simulink model "RETRO_IFF_NON_LIN"  (R2021a)
settings: Solver=VariableStepAuto  StartTime=0.0  StopTime=300  RelTol=1e-3
model workspace (MATLAB code in the model file):
  | Kab=14;
  | Fa=4;
  | Kba=10;
  | Fb=4;
  | Kca=8;
  | Kcb=3.2;
  | Kcd=6;
  | Fc=2;
  | Kdc=6;
  | Fd=0.5;
  | Kia=5;
  | Fa=6;
  | In=0.3;
  | x_star=[0.25;0.625;0.0833;0];
settings Model: Creator=priya  LastModifiedBy=Priyan_PC
settings SolverCC: AlgebraicLoopSolver=TrustRegion
settings DebuggingCC: SFMachineParentedDataDiag=warning

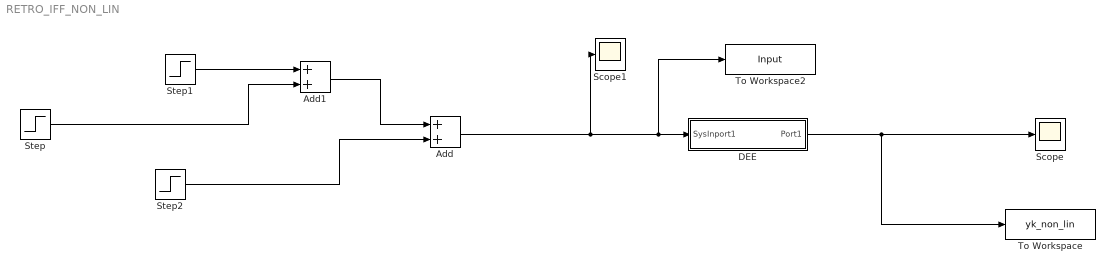
== system RETRO_IFF_NON_LIN ==
  Add : Sum
  Add1 : Sum
  DEE : Subsystem  mask(Differential Equation Editor (DEE)){}
      settings: OpenFcn=diffeqed
      mask Display: disp('Differential Equation\n Editor')
  Scope : Scope
  Scope1 : Scope
  Step : Step  Time=75  After=0.15  SampleTime=0
  Step1 : Step  Time=0  Before=0.3  After=0.5  SampleTime=0
  Step2 : Step  Time=150  After=0.15  SampleTime=0
  To Workspace : ToWorkspace  VariableName=yk_non_lin  SampleTime=-1
  To Workspace2 : ToWorkspace  VariableName=Input  SampleTime=-1
  wires:
  Step1/1 -> Add1/1
  Step/1 -> Add1/2
  Step2/1 -> Add/2
  Add1/1 -> Add/1
  Add/1 -> To Workspace2/1, DEE/1(SysInport1), Scope1/1
  DEE/1(Port1) -> To Workspace/1, Scope/1

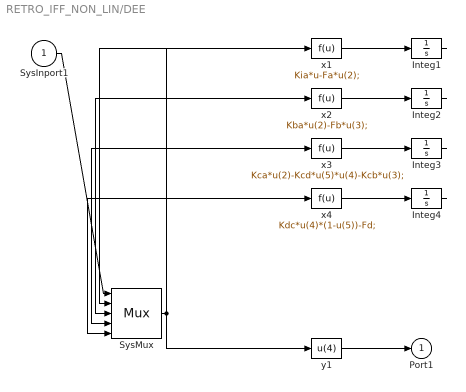
== system RETRO_IFF_NON_LIN/DEE ==
  SysInport1 : Inport
  Integ1 : Integrator  InitialCondition=x_star(1)
  Integ2 : Integrator  InitialCondition=x_star(2)
  Integ3 : Integrator  InitialCondition=x_star(3)
  Integ4 : Integrator  InitialCondition=x_star(4)
  SysMux : Mux  Inputs=5
  x1 : Fcn  Expr=Kia*u-Fa*u(2);
  x2 : Fcn  Expr=Kba*u(2)-Fb*u(3);
  x3 : Fcn  Expr=Kca*u(2)-Kcd*u(5)*u(4)-Kcb*u(3);
  x4 : Fcn  Expr=Kdc*u(4)*(1-u(5))-Fd;
  y1 : Fcn  Expr=u(4)
  Port1 : Outport
  wires:
  SysInport1/1 -> SysMux/1
  SysMux/1 -> x1/1, x2/1, x3/1, x4/1, y1/1
  x1/1 -> Integ1/1
  Integ1/1 -> SysMux/2
  x2/1 -> Integ2/1
  Integ2/1 -> SysMux/3
  x3/1 -> Integ3/1
  Integ3/1 -> SysMux/4
  x4/1 -> Integ4/1
  Integ4/1 -> SysMux/5
  y1/1 -> Port1/1
